simulink model "Triac_Pilot_V1"  (R2020a)
settings: Solver=FixedStepAuto  StartTime=0.0  StopTime=10.0  FixedStep=0.0001  RelTol=1e-3
undefined symbols (not defined in the file): DiscIntNeverNeededParam
settings Model: Creator=BEDNASA  LastModifiedBy=BEDNASA

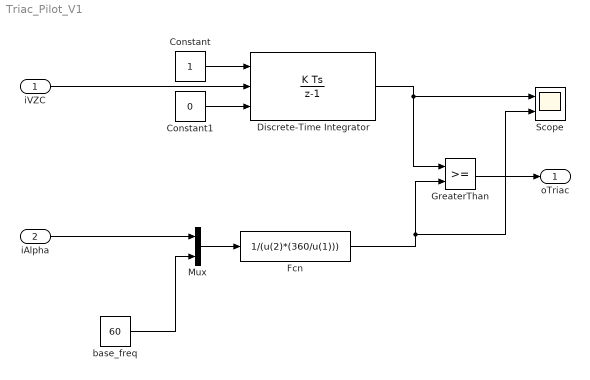
== system Triac_Pilot_V1 ==
  iVZC : Inport
  iAlpha : Inport  Port=2
  Constant : Constant
  Constant1 : Constant  Value=0
  Discrete-Time Integrator : DiscreteIntegrator  ExternalReset=either  InitialConditionSource=external  SampleTime=-1  ICPrevOutput=DiscIntNeverNeededParam  ICPrevScaledInput=DiscIntNeverNeededParam
  Fcn : Fcn  Expr=1/(u(2)*(360/u(1)))
  GreaterThan : RelationalOperator  OutDataTypeStr=boolean  RndMeth=Simplest
  Mux : Mux  Inputs=2
  Scope : Scope  NumInputPorts=2
  base_freq : Constant  Value=60  SampleTime=-1
  oTriac : Outport
  wires:
  GreaterThan/1 -> oTriac/1
  Mux/1 -> Fcn/1
  Fcn/1 -> Scope/2, GreaterThan/2
  base_freq/1 -> Mux/2
  iAlpha/1 -> Mux/1
  Constant/1 -> Discrete-Time Integrator/1
  Constant1/1 -> Discrete-Time Integrator/3
  iVZC/1 -> Discrete-Time Integrator/2
  Discrete-Time Integrator/1 -> GreaterThan/1, Scope/1
